simulink model "Copy_of_ModeStatAndRsp"  (R2018b)
settings: Solver=FixedStepDiscrete  StartTime=0.0  StopTime=10.0  FixedStep=0.01  RelTol=1e-3
undefined symbols (not defined in the file): c_RecvL, c_RecvLR, c_RecvR, IfVeSMSeStNumConfig, KeSMSbMdChime2Enable_Val, KeSMSbSRSPosNumConfig_Val, KeSMSuChmReqDurnTm_Val, KeSMSuChmReqIntlTm_Val, KeSMSuRspStatHldTm_Val, MdRspLocal1, MdTp1, ModeNum, PowerMode1, SrcReqTp1, srsconvert
libraries: RspLib x47, simulink x1
(part 6 of 8)

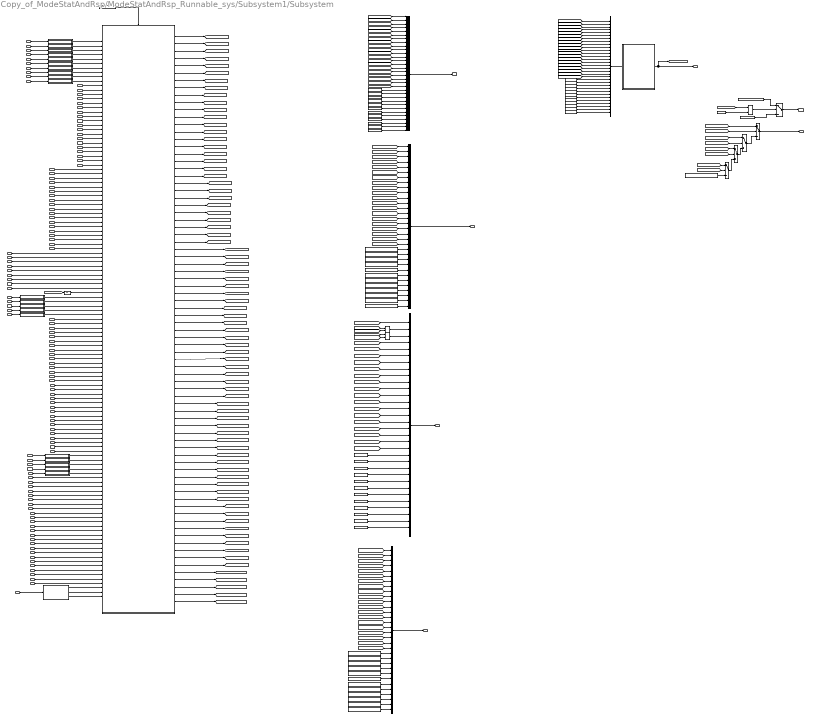
== system Copy_of_ModeStatAndRsp/ModeStatAndRsp_Runnable_sys/Subsystem1/Subsystem ==
  note: **信号已使用不被使用，暂时保留
  acsExtMdReq : Inport
  acsEntyMdReq : Inport  Port=2
  LtVipMdReq : Inport  Port=3
  RtVipMdReq : Inport  Port=4
  AllVipMdReq : Inport  Port=5
  LtLugMdReq : Inport  Port=6
  RtLugMdReq : Inport  Port=7
  AllLugMdReq : Inport  Port=8
  LtRcvyMdReq : Inport  Port=9
  RtRcvyMdReq : Inport  Port=10
  CommCond : Inport  Port=11
  CommExitCond : Inport  Port=12
  CommExitCondwithSpeed : Inport  Port=13
  isAcsMdEntryDoneOK : Inport  Port=14
  isAcsMdExtDoneOK : Inport  Port=15
  isLfLugDoneOK : Inport  Port=16
  isLfRecoveryDoneOK : Inport  Port=17
  isLfVipDoneOK : Inport  Port=18
  isRtLugDoneOK : Inport  Port=19
  isRtRecoveryDoneOK : Inport  Port=20
  isRtVipDoneOK : Inport  Port=21
  isAcsMdEntryDoneFailed : Inport  Port=22
  isAcsMdExtDoneFailed : Inport  Port=23
  isLfLugDoneFailed : Inport  Port=24
  isLfRecoveryDoneFailed : Inport  Port=25
  isLfVipDoneFailed : Inport  Port=26
  isRtLugDoneFailed : Inport  Port=27
  isRtRecoveryDoneFailed : Inport  Port=28
  isRtVipDoneFailed : Inport  Port=29
  SwIntAcsEnty : Inport  Port=30
  SwIntAcsExt : Inport  Port=31
  SwIntLfVip : Inport  Port=32
  SwIntRtVip : Inport  Port=33
  SwIntLfLug : Inport  Port=34
  SwIntRtLug : Inport  Port=35
  SwIntLfRcvy : Inport  Port=36
  SwIntRtRcvy : Inport  Port=37
  SwIntAllLug : Inport  Port=38
  SoftIntAcsExt : Inport  Port=39
  SoftIntAcsEnty : Inport  Port=40
  SoftIntLfVip : Inport  Port=41
  SoftIntRtVip : Inport  Port=42
  SoftIntLfLug : Inport  Port=43
  SoftIntRtLug : Inport  Port=44
  SoftIntLfRcvy : Inport  Port=45
  SoftIntRtRcvy : Inport  Port=46
  SoftIntAllVip : Inport  Port=47
  SoftIntAllLug : Inport  Port=48
  acsExtMdSrcTp : Inport  Port=49
  acsEntyMdSrcTp : Inport  Port=50
  LtVipSrcReqTp : Inport  Port=51
  RtVipSrcReqTp : Inport  Port=52
  LtLugSrcReqTp : Inport  Port=53
  RtLugSrcReqTp : Inport  Port=54
  LtRcvySrcReqTp : Inport  Port=55
  RtRcvySrcReqTp : Inport  Port=56
  AllLugSrcReqTp_Val : Inport  Port=57
  StNumConfig : Inport  Port=58
  INTMMdReq : Inport  Port=59
  LfFamlyReq : Inport  Port=60
  LfLyMdReq : Inport  Port=61
  RtFamlyMdReq : Inport  Port=62
  RtLyMdReq : Inport  Port=63
  INTMSrcReqTp : Inport  Port=64
  LfFamlySrcReqTp : Inport  Port=65
  LfLySrcReqTp : Inport  Port=66
  RtFamlySrcReqTp : Inport  Port=67
  RtLySrcReqTp : Inport  Port=68
  SoftIntINTM : Inport  Port=69
  SoftIntLfFamly : Inport  Port=70
  SoftIntLfLy : Inport  Port=71
  SoftIntRtFamly : Inport  Port=72
  SoftIntRtLy : Inport  Port=73
  SwIntINTM : Inport  Port=74
  SwIntLfFamly : Inport  Port=75
  SwIntLfLy : Inport  Port=76
  SwIntRtFamly : Inport  Port=77
  SwIntRtLy : Inport  Port=78
  isINTMDoneOK : Inport  Port=79
  isFamlyLDoneOK : Inport  Port=80
  isFamlyRDoneOK : Inport  Port=81
  isLfLyDoneOK : Inport  Port=82
  isRtLyDoneOK : Inport  Port=83
  isINTMDoneFailed : Inport  Port=84
  isFamlyLDoneFailed : Inport  Port=85
  isFamlyRDoneFailed : Inport  Port=86
  isLfLyDoneFailed : Inport  Port=87
  isRtLyDoneFailed : Inport  Port=88
  AllVipSrcReqTp : Inport  Port=89
  LugMdLtAvl_Val_read : Inport  Port=90
  LugMdRtAvl_Val_read : Inport  Port=91
  VipMdLtAvl_Val_read : Inport  Port=92
  VipMdRtAvl_Val_read : Inport  Port=93
  SwIntAllVip : Inport  Port=94
  IntimacyRtMdReq_Val_read : Inport  Port=95
  IntimacyRtMdSrcTp_Val_read : Inport  Port=96
  isINTMRDoneFailed_Val_read : Inport  Port=97
  isINTMRDoneOK_Val_read : Inport  Port=98
  isLgrstCloseLDoneFailed_Val_read : Inport  Port=99
  isLgrstCloseLDoneOK_Val_read : Inport  Port=100
  isLgrstCloseRDoneFailed_Val_read : Inport  Port=101
  isLgrstCloseRDoneOK_Val_read : Inport  Port=102
  isLgrstOpenLDoneFailed_Val_read : Inport  Port=103
  isLgrstOpenLDoneOK_Val_read : Inport  Port=104
  isLgrstOpenRDoneFailed_Val_read : Inport  Port=105
  isLgrstOpenRDoneOK_Val_read : Inport  Port=106
  LgrstCloseLtMdReq_Val_read : Inport  Port=107
  LgrstCloseLtSrcReqTp_Val_read : Inport  Port=108
  LgrstCloseRtMdReq_Val_read : Inport  Port=109
  LgrstCloseRtSrcReqTp_Val_read : Inport  Port=110
  LgrstOpenLtMdReq_Val_read : Inport  Port=111
  LgrstOpenLtSrcReqTp_Val_read : Inport  Port=112
  LgrstOpenRtMdReq_Val_read : Inport  Port=113
  LgrstOpenRtSrcReqTp_Val_read : Inport  Port=114
  SoftIntIntimacyRt_Val_read : Inport  Port=115
  SoftIntLgrstCloseLt_Val_read : Inport  Port=116
  SoftIntLgrstCloseRt_Val_read : Inport  Port=117
  SoftIntLgrstOpenLt_Val_read : Inport  Port=118
  SoftIntLgrstOpenRt_Val_read : Inport  Port=119
  SwIntIntimacyRt_Val_read : Inport  Port=120
  SwIntLgrstCloseLt_Val_read : Inport  Port=121
  SwIntLgrstCloseRt_Val_read : Inport  Port=122
  SwIntLgrstOpenLt_Val_read : Inport  Port=123
  SwIntLgrstOpenRt_Val_read : Inport  Port=124
  Bus Creator{,1,3..4} (4 alike) : BusCreator  Inputs=32
  Chart : Stateflow chart  TreatAsAtomicUnit=on
  Chart2 : Stateflow chart  TreatAsAtomicUnit=on
  Constant{7,9..18,36..37} (13 alike) : Constant  Value=SrcReqTp1.SrcReqTp_None  OutDataTypeStr=Enum:SrcReqTp1
  Constant{19..30} (12 alike) : Constant  Description=_SGMK226P2.FCMD.000_369_  Value=0  OutDataTypeStr=boolean
  Constant3 : Constant  Value=MdTp1.MdTp_EzeEntry  OutDataTypeStr=Enum:MdTp1
  Constant{38..49} (12 alike) : Constant  Value=MdRspLocal1.MdRsp_None  OutDataTypeStr=Enum: MdRspLocal1
  Constant5 : Constant  Value=0  OutDataTypeStr=uint32
  Constant{56..67,73..84} (24 alike) : Constant  Value=0  OutDataTypeStr=boolean
  Constant6 : Constant  Value=MdTp1.MdTp_None  OutDataTypeStr=Enum:MdTp1
  Function-Call Generator : simulink/Ports & Subsystems/Function-Call Generator  sample_time=-1  numberOfIterations=2
  HasChangeToTrue : Subsystem
  HasChangeToTrue1 : Subsystem
  HasChangeToTrue10 : Subsystem
  HasChangeToTrue11 : Subsystem
  HasChangeToTrue12 : Subsystem
  HasChangeToTrue13 : Subsystem
  HasChangeToTrue14 : Subsystem
  HasChangeToTrue15 : Subsystem
  HasChangeToTrue16 : Subsystem
  HasChangeToTrue17 : Subsystem
  HasChangeToTrue18 : Subsystem
  HasChangeToTrue19 : Subsystem
  HasChangeToTrue2 : Subsystem
  HasChangeToTrue3 : Subsystem
  HasChangeToTrue4 : Subsystem
  HasChangeToTrue5 : Subsystem
  HasChangeToTrue6 : Subsystem
  HasChangeToTrue7 : Subsystem
  HasChangeToTrue8 : Subsystem
  HasChangeToTrue9 : Subsystem
  Mux11 : Mux  Inputs=32
  OR : Logic  Operator=OR  AllPortsSameDT=off  OutDataTypeStr=boolean
  OR1 : Logic  Operator=OR  AllPortsSameDT=off  OutDataTypeStr=boolean
  Relational Operator : RelationalOperator  Operator=>  OutDataTypeStr=boolean  RndMeth=Simplest
  StNumChk : Subsystem
  Switch{,1..4} (5 alike) : Switch  Criteria=u2 > Threshold
  Unit Delay9 : UnitDelay  SampleTime=-1
  oModeState : Outport
  ModeSrcTpLt : Outport  Port=2  VectorParamsAs1DForOutWhenUnconnected=on
  ModeState32 : Outport  Port=3
  MdStateBus : Outport  Port=4
  MdBsy : Outport  Port=5
  MdSrcTp : Outport  Port=6
  MdRsp : Outport  Port=7
  wires:
  SwIntRtVip/1 -> Chart/33(SwIntRtVip)
  isRtLugDoneOK/1 -> Chart/19(iIsRtLugDoneOK)
  SoftIntAcsEnty/1 -> Chart/40(SoftIntAcsEnty)
  SoftIntLfRcvy/1 -> Chart/45(SoftIntLfRcvy)
  SoftIntRtRcvy/1 -> Chart/46(SoftIntRtRcvy)
  isRtRecoveryDoneFailed/1 -> Chart/28(iIsRtRecoveryDoneFailed)
  isAcsMdExtDoneFailed/1 -> Chart/23(iIsAcsMdExtDoneFailed)
  isAcsMdEntryDoneOK/1 -> Chart/14(iIsAcsMdEntryDoneOK)
  SwIntAcsExt/1 -> Chart/31(SwIntAcsExt)
  SoftIntRtLug/1 -> Chart/44(SoftIntRtLug)
  SoftIntRtVip/1 -> Chart/42(SoftIntRtVip)
  isRtRecoveryDoneOK/1 -> Chart/20(iIsRtRecoveryDoneOK)
  SoftIntAllLug/1 -> Chart/48(SoftIntAllLug)
  isAcsMdEntryDoneFailed/1 -> Chart/22(iIsAcsMdEntryDoneFailed)
  SwIntRtRcvy/1 -> Chart/37(SwIntRtRcvy)
  isLfLugDoneFailed/1 -> Chart/24(iIsLtLugDoneFailed)
  CommExitCond/1 -> Chart/12(CommExitCond)
  isLfVipDoneOK/1 -> Chart/18(iIsLtVipDoneOK)
  CommCond/1 -> Chart/11(CommCond)
  SwIntRtLug/1 -> Chart/35(SwIntRtLug)
  SoftIntAllVip/1 -> Chart/47(SoftIntAllVip)
  isAcsMdExtDoneOK/1 -> Chart/15(iIsAcsMdExtDoneOK)
  isLfLugDoneOK/1 -> Chart/16(iIsLtLugDoneOK)
  SoftIntAcsExt/1 -> Chart/39(SoftIntAcsExt)
  SwIntAllLug/1 -> Chart/38(SwIntAllLug)
  isLfRecoveryDoneOK/1 -> Chart/17(iIsLtRecoveryDoneOK)
  isRtVipDoneOK/1 -> Chart/21(iIsRtVipDoneOK)
  isRtLugDoneFailed/1 -> Chart/27(iIsRtLugDoneFailed)
  SoftIntLfVip/1 -> Chart/41(SoftIntLfVip)
  isLfRecoveryDoneFailed/1 -> Chart/25(iIsLtRecoveryDoneFailed)
  SwIntLfRcvy/1 -> Chart/36(SwIntLfRcvy)
  isLfVipDoneFailed/1 -> Chart/26(iIsLtVipDoneFailed)
  isRtVipDoneFailed/1 -> Chart/29(iIsRtVipDoneFailed)
  SwIntLfLug/1 -> Chart/34(SwIntLfLug)
  SoftIntLfLug/1 -> Chart/43(SoftIntLfLug)
  SwIntAcsEnty/1 -> Chart/30(SwIntAcsEnty)
  SwIntLfVip/1 -> Chart/32(SwIntLfVip)
  CommExitCondwithSpeed/1 -> Chart/13(CommExitCondwithSpeed)
  [LgrstOpenR_En] -> Mux11/18
  Mux11/1 -> Chart2/1(ModeArray)
  Constant20/1 -> Mux11/22
  Constant26/1 -> Mux11/28
  [LgrstCloseL_En] -> Mux11/17
  [RecoveryR_En] -> Mux11/13
  [FAMLY_R_En] -> Mux11/6
  [LgrstCloseR_En] -> Mux11/19
  [INTM_En] -> Mux11/5
  [INTMR_En] -> Mux11/20
  [LgrstOpenL_En] -> Mux11/16
  Constant29/1 -> Mux11/31
  [RecoveryL_En] -> Mux11/11
  Constant28/1 -> Mux11/30
  Constant27/1 -> Mux11/29
  [VIPR_En] -> Mux11/12
  [LugL_En] -> Mux11/8
  [VIPAll_En] -> Mux11/2
  Constant22/1 -> Mux11/24
  Constant24/1 -> Mux11/26
  [LyL_En] -> Mux11/14
  [EZE_En] -> Mux11/1
  [LugAll_En] -> Mux11/3
  [FAMLY_L_En] -> Mux11/7
  [LugR_En] -> Mux11/9
  Constant30/1 -> Mux11/32
  Constant23/1 -> Mux11/25
  Constant19/1 -> Mux11/21
  [EZQ_En] -> Mux11/4
  [VIPL_En] -> Mux11/10
  Constant25/1 -> Mux11/27
  Constant21/1 -> Mux11/23
  [LyR_En] -> Mux11/15
  Chart/11(RecoveryL_En) -> [RecoveryL_En]
  Chart/10(VIPL_En) -> [VIPL_En]
  Chart/12(VIPR_En) -> [VIPR_En]
  Chart/9(LugR_En) -> [LugR_En]
  Chart/13(RecoveryR_En) -> [RecoveryR_En]
  Chart/8(LugL_En) -> [LugL_En]
  Chart/14(LyL_En) -> [LyL_En]
  Chart/7(FAMLY_L_En) -> [FAMLY_L_En]
  Chart/15(LyR_En) -> [LyR_En]
  Chart/6(FAMLY_R_En) -> [FAMLY_R_En]
  Chart/5(INTM_En) -> [INTM_En]
  Chart/4(EZQ_En) -> [EZQ_En]
  Chart/3(LugAll_En) -> [LugAll_En]
  Chart/2(VIPAll_En) -> [VIPAll_En]
  Chart2/1(ModeState32) -> [ModeState32], ModeState32/1
  [ModeState32] -> Relational Operator/1
  Constant5/1 -> Relational Operator/2
  Relational Operator/1 -> Switch/2
  Constant3/1 -> Switch/1
  Switch/1 -> oModeState/1
  Constant6/1 -> Switch/3
  Chart/21(ModeSrcTpAllLug) -> [ModeSrcTpAllLug]
  Chart/22(ModeSrcTpEZE) -> [ModeSrcTpEZE]
  Chart/23(ModeSrcTpEZQ) -> [ModeSrcTpEZQ]
  Chart/24(ModeSrcTpLtLug) -> [ModeSrcTpLtLug]
  Chart/25(ModeSrcTpLtRecovery) -> [ModeSrcTpLtRecovery]
  Chart/26(ModeSrcTpLtVIP) -> [ModeSrcTpLtVIP]
  Chart/27(ModeSrcTpRtLug) -> [ModeSrcTpRtLug]
  Chart/28(ModeSrcTpRtRecovery) -> [ModeSrcTpRtRecovery]
  Chart/29(ModeSrcTpRtVIP) -> [ModeSrcTpRtVIP]
  Chart/1(EZE_En) -> [EZE_En]
  [ModeState32] -> Unit Delay9/1
  Unit Delay9/1 -> Chart/58(modestate32)
  Switch1/1 -> ModeSrcTpLt/1
  [EZE_En] -> Switch1/2
  [ModeSrcTpEZE] -> Switch1/1
  Switch2/1 -> Switch1/3
  [EZQ_En] -> Switch2/2
  [ModeSrcTpEZQ] -> Switch2/1
  Switch3/1 -> Switch2/3
  [VIPAll_En] -> Switch3/2
  [ModeSrcTpALLVIP] -> Switch3/1
  Switch4/1 -> Switch3/3
  [LugAll_En] -> Switch4/2
  [ModeSrcTpAllLug] -> Switch4/1
  Constant7/1 -> Switch4/3
  SoftIntINTM/1 -> Chart/64(SoftIntINTM)
  SoftIntLfFamly/1 -> Chart/65(SoftIntLfFamly)
  SoftIntLfLy/1 -> Chart/66(SoftIntLfLy)
  SoftIntRtFamly/1 -> Chart/67(SoftIntRtFamly)
  SoftIntRtLy/1 -> Chart/68(SoftIntRtLy)
  SwIntINTM/1 -> Chart/69(SwIntINTM)
  SwIntLfFamly/1 -> Chart/70(SwIntLfFamly)
  SwIntLfLy/1 -> Chart/71(SwIntLfLy)
  SwIntRtFamly/1 -> Chart/72(SwIntRtFamly)
  SwIntRtLy/1 -> Chart/73(SwIntRtLy)
  isINTMDoneOK/1 -> Chart/74(isINTMDoneOK)
  isFamlyLDoneOK/1 -> Chart/75(isFamlyLDoneOK)
  isFamlyRDoneOK/1 -> Chart/76(isFamlyRDoneOK)
  isLfLyDoneOK/1 -> Chart/77(isLfLyDoneOK)
  isRtLyDoneOK/1 -> Chart/78(isRtLyDoneOK)
  isINTMDoneFailed/1 -> Chart/79(isINTMDoneFailed)
  isFamlyLDoneFailed/1 -> Chart/80(isFamlyLDoneFailed)
  isFamlyRDoneFailed/1 -> Chart/81(isFamlyRDoneFailed)
  isLfLyDoneFailed/1 -> Chart/82(isLfLyDoneFailed)
  isRtLyDoneFailed/1 -> Chart/83(isRtLyDoneFailed)
  Chart/50(ModeSrcTpALLVIP) -> [ModeSrcTpALLVIP]
  Chart/52(EZQStBsy) -> [EZQStBsy]
  Chart/51(EZEStBsy) -> [EZEStBsy]
  Chart/53(VIPLStBsy) -> [VIPLStBsy]
  Chart/54(VIPRStBsy) -> [VIPRStBsy]
  Chart/55(RecoveryLStBsy) -> [RecoveryLStBsy]
  Chart/56(RecoveryRStBsy) -> [RecoveryRStBsy]
  Chart/57(LugLStBsy) -> [LugLStBsy]
  Chart/58(LugRStBsy) -> [LugRStBsy]
  Chart/59(FamlyLBsy) -> [FamilyLStBsy]
  Chart/60(FamlyRBsy) -> [FamilyRStBsy]
  Chart/61(INTMBsy) -> [INTMBsy]
  Chart/62(LyLBsy) -> [LyLBsy]
  Chart/63(LyRBsy) -> [LyRBsy]
  LugMdLtAvl_Val_read/1 -> Chart/90(LugMdLtAvl)
  LugMdRtAvl_Val_read/1 -> Chart/91(LugMdRtAvl)
  VipMdLtAvl_Val_read/1 -> Chart/92(VipMdLtAvl)
  VipMdRtAvl_Val_read/1 -> Chart/93(VipMdRtAvl)
  SwIntAllVip/1 -> Chart/94(SwIntAllVip)
  Function-Call Generator/1 -> Chart/Trigger
  acsExtMdReq/1 -> HasChangeToTrue/1(In1)
  acsEntyMdReq/1 -> HasChangeToTrue1/1(In1)
  LtVipMdReq/1 -> HasChangeToTrue2/1(In1)
  RtVipMdReq/1 -> HasChangeToTrue3/1(In1)
  AllVipMdReq/1 -> HasChangeToTrue4/1(In1)
  LtLugMdReq/1 -> HasChangeToTrue5/1(In1)
  RtLugMdReq/1 -> HasChangeToTrue6/1(In1)
  AllLugMdReq/1 -> HasChangeToTrue7/1(In1)
  LtRcvyMdReq/1 -> HasChangeToTrue8/1(In1)
  RtRcvyMdReq/1 -> HasChangeToTrue9/1(In1)
  acsExtMdSrcTp/1 -> Chart/49(acsExtMdSrcTp)
  acsEntyMdSrcTp/1 -> Chart/50(acsEntyMdSrcTp)
  LtVipSrcReqTp/1 -> Chart/51(LtVipSrcReqTp)
  RtVipSrcReqTp/1 -> Chart/52(RtVipSrcReqTp)
  LtLugSrcReqTp/1 -> Chart/53(LtLugSrcReqTp)
  RtLugSrcReqTp/1 -> Chart/54(RtLugSrcReqTp)
  LtRcvySrcReqTp/1 -> Chart/55(LtRcvySrcReqTp)
  RtRcvySrcReqTp/1 -> Chart/56(RtRcvySrcReqTp)
  AllLugSrcReqTp_Val/1 -> Chart/57(AllLugSrcReqTp)
  INTMMdReq/1 -> HasChangeToTrue10/1(In1)
  LfFamlyReq/1 -> HasChangeToTrue11/1(In1)
  LfLyMdReq/1 -> HasChangeToTrue12/1(In1)
  RtFamlyMdReq/1 -> HasChangeToTrue13/1(In1)
  RtLyMdReq/1 -> HasChangeToTrue14/1(In1)
  INTMSrcReqTp/1 -> Chart/84(INTMSrcReqTp)
  LfFamlySrcReqTp/1 -> Chart/85(LfFamlySrcReqTp)
  LfLySrcReqTp/1 -> Chart/86(LfLySrcReqTp)
  RtFamlySrcReqTp/1 -> Chart/87(RtFamlySrcReqTp)
  RtLySrcReqTp/1 -> Chart/88(RtLySrcReqTp)
  AllVipSrcReqTp/1 -> Chart/89(AllVipSrcReqTp)
  HasChangeToTrue/1(Out1) -> Chart/1(acsExtMdReq)
  HasChangeToTrue1/1(Out1) -> Chart/2(acsEntyMdReq)
  HasChangeToTrue2/1(Out1) -> Chart/3(LtVipMdReq)
  HasChangeToTrue3/1(Out1) -> Chart/4(RtVipMdReq)
  HasChangeToTrue4/1(Out1) -> Chart/5(AllVipMdReq)
  HasChangeToTrue5/1(Out1) -> Chart/6(LtLugMdReq)
  HasChangeToTrue6/1(Out1) -> Chart/7(RtLugMdReq)
  HasChangeToTrue7/1(Out1) -> Chart/8(AllLugMdReq)
  HasChangeToTrue8/1(Out1) -> Chart/9(LtRcvyMdReq)
  HasChangeToTrue9/1(Out1) -> Chart/10(RtRcvyMdReq)
  HasChangeToTrue10/1(Out1) -> Chart/59(INTMMdReq)
  HasChangeToTrue11/1(Out1) -> Chart/60(LfFamlyMdReq)
  HasChangeToTrue12/1(Out1) -> Chart/61(LfLyMdReq)
  HasChangeToTrue13/1(Out1) -> Chart/62(RtFamlyMdReq)
  HasChangeToTrue14/1(Out1) -> Chart/63(RtLyMdReq)
  Chart/16(LgrstOpenL_En) -> [LgrstOpenL_En]
  Chart/17(LgrstCloseL_En) -> [LgrstCloseL_En]
  Chart/18(LgrstOpenR_En) -> [LgrstOpenR_En]
  Chart/19(LgrstCloseR_En) -> [LgrstCloseR_En]
  Chart/20(INTMR_En) -> [INTMR_En]
  IntimacyRtMdReq_Val_read/1 -> HasChangeToTrue15/1(In1)
  LgrstCloseLtMdReq_Val_read/1 -> HasChangeToTrue16/1(In1)
  LgrstCloseRtMdReq_Val_read/1 -> HasChangeToTrue17/1(In1)
  LgrstOpenLtMdReq_Val_read/1 -> HasChangeToTrue18/1(In1)
  LgrstOpenRtMdReq_Val_read/1 -> HasChangeToTrue19/1(In1)
  IntimacyRtMdSrcTp_Val_read/1 -> Chart/100(INTMRSrcReqTp)
  LgrstCloseLtSrcReqTp_Val_read/1 -> Chart/101(LgrstCloseLtSrcReqTp)
  LgrstCloseRtSrcReqTp_Val_read/1 -> Chart/102(LgrstCloseRtSrcReqTp)
  LgrstOpenLtSrcReqTp_Val_read/1 -> Chart/103(LgrstOpenLtSrcReqTp)
  LgrstOpenRtSrcReqTp_Val_read/1 -> Chart/104(LgrstOpenRtSrcReqTp)
  isINTMRDoneFailed_Val_read/1 -> Chart/105(isINTMRDoneFailed)
  isLgrstCloseLDoneFailed_Val_read/1 -> Chart/106(isLgrstCloseLDoneFailed)
  isLgrstCloseRDoneFailed_Val_read/1 -> Chart/107(isLgrstCloseRDoneFailed)
  isLgrstOpenLDoneFailed_Val_read/1 -> Chart/108(isLgrstOpenLDoneFailed)
  isLgrstOpenRDoneFailed_Val_read/1 -> Chart/109(isLgrstOpenRDoneFailed)
  isINTMRDoneOK_Val_read/1 -> Chart/110(isINTMRDoneOK)
  isLgrstCloseLDoneOK_Val_read/1 -> Chart/111(isLgrstCloseLDoneOK)
  isLgrstCloseRDoneOK_Val_read/1 -> Chart/112(isLgrstCloseRDoneOK)
  isLgrstOpenLDoneOK_Val_read/1 -> Chart/113(isLgrstOpenLDoneOK)
  isLgrstOpenRDoneOK_Val_read/1 -> Chart/114(isLgrstOpenRDoneOK)
  SoftIntIntimacyRt_Val_read/1 -> Chart/115(SoftIntINTMR)
  SoftIntLgrstCloseLt_Val_read/1 -> Chart/116(SoftIntLgrstCloseLt)
  SoftIntLgrstCloseRt_Val_read/1 -> Chart/117(SoftIntLgrstCloseRt)
  SoftIntLgrstOpenLt_Val_read/1 -> Chart/118(SoftIntLgrstOpenLt)
  SoftIntLgrstOpenRt_Val_read/1 -> Chart/119(SoftIntLgrstOpenRt)
  SwIntIntimacyRt_Val_read/1 -> Chart/120(SwIntINTMR)
  SwIntLgrstCloseLt_Val_read/1 -> Chart/121(SwIntLgrstCloseLt)
  SwIntLgrstCloseRt_Val_read/1 -> Chart/122(SwIntLgrstCloseRt)
  SwIntLgrstOpenLt_Val_read/1 -> Chart/123(SwIntLgrstOpenLt)
  SwIntLgrstOpenRt_Val_read/1 -> Chart/124(SwIntLgrstOpenRt)
  HasChangeToTrue15/1(Out1) -> Chart/95(INTMRMdReq)
  HasChangeToTrue16/1(Out1) -> Chart/96(LgrstCloseLtMdReq)
  HasChangeToTrue17/1(Out1) -> Chart/97(LgrstCloseRtMdReq)
  HasChangeToTrue18/1(Out1) -> Chart/98(LgrstOpenLtMdReq)
  HasChangeToTrue19/1(Out1) -> Chart/99(LgrstOpenRtMdReq)
  Chart/78(INTMRBsy) -> [INTMRBsy]
  Chart/77(LgrstCloseRBsy) -> [LgrstCloseRBsy]
  Chart/75(LgrstCloseLBsy) -> [LgrstCloseLBsy]
  Chart/76(LgrstOpenRBsy) -> [LgrstOpenRBsy]
  Chart/74(LgrstOpenLBsy) -> [LgrstOpenLBsy]
  [LgrstCloseR_En] -> Bus Creator3/19  "Md19_En"
  [LgrstOpenL_En] -> Bus Creator3/16  "Md16_En"
  [EZE_En] -> Bus Creator3/1  "Md1_En"
  [LugL_En] -> Bus Creator3/8  "Md8_En"
  Constant67/1 -> Bus Creator3/32  "Md32_En"
  [FAMLY_L_En] -> Bus Creator3/7  "Md7_En"
  [RecoveryR_En] -> Bus Creator3/13  "Md13_En"
  Constant61/1 -> Bus Creator3/26  "Md26_En"
  [FAMLY_R_En] -> Bus Creator3/6  "Md6_En"
  [LgrstOpenR_En] -> Bus Creator3/18  "Md18_En"
  Constant57/1 -> Bus Creator3/22  "Md22_En"
  Constant59/1 -> Bus Creator3/24  "Md24_En"
  Constant56/1 -> Bus Creator3/21  "Md21_En"
  [LyR_En] -> Bus Creator3/15  "Md15_En"
  Constant65/1 -> Bus Creator3/30  "Md30_En"
  Constant64/1 -> Bus Creator3/29  "Md29_En"
  Constant66/1 -> Bus Creator3/31  "Md31_En"
  Constant62/1 -> Bus Creator3/27  "Md27_En"
  Constant58/1 -> Bus Creator3/23  "Md23_En"
  [VIPAll_En] -> Bus Creator3/2  "Md2_En"
  [INTMR_En] -> Bus Creator3/20  "Md20_En"
  [VIPL_En] -> Bus Creator3/10  "Md10_En"
  [LgrstCloseL_En] -> Bus Creator3/17  "Md17_En"
  [LyL_En] -> Bus Creator3/14  "Md14_En"
  [RecoveryL_En] -> Bus Creator3/11  "Md11_En"
  [LugR_En] -> Bus Creator3/9  "Md9_En"
  Constant60/1 -> Bus Creator3/25  "Md25_En"
  [LugAll_En] -> Bus Creator3/3  "Md3_En"
  [INTM_En] -> Bus Creator3/5  "Md5_En"
  [EZQ_En] -> Bus Creator3/4  "Md4_En"
  Constant63/1 -> Bus Creator3/28  "Md28_En"
  [VIPR_En] -> Bus Creator3/12  "Md12_En"
  Bus Creator3/1 -> MdStateBus/1
  Constant76/1 -> Bus Creator4/24  "Md24Exit"
  [LyRBsy] -> Bus Creator4/15  "Md15Exit"
  Constant82/1 -> Bus Creator4/30  "Md30Exit"
  Constant78/1 -> Bus Creator4/26  "Md26Exit"
  Constant80/1 -> Bus Creator4/28  "Md28Exit"
  [EZEStBsy] -> Bus Creator4/1  "Md1Exit"
  Constant79/1 -> Bus Creator4/27  "Md27Exit"
  [LugLStBsy] -> Bus Creator4/8  "Md8Exit"
  Constant81/1 -> Bus Creator4/29  "Md29Exit"
  Constant77/1 -> Bus Creator4/25  "Md25Exit"
  Constant75/1 -> Bus Creator4/23  "Md23Exit"
  [INTMRBsy] -> Bus Creator4/20  "Md20Exit"
  Constant73/1 -> Bus Creator4/21  "Md21Exit"
  [LgrstCloseRBsy] -> Bus Creator4/19  "Md19Exit"
  [FamilyRStBsy] -> Bus Creator4/6  "Md6Exit"
  [LyLBsy] -> Bus Creator4/14  "Md14Exit"
  Constant83/1 -> Bus Creator4/31  "Md31Exit"
  [FamilyLStBsy] -> Bus Creator4/7  "Md7Exit"
  [LugLStBsy] -> OR1/1
  [RecoveryRStBsy] -> Bus Creator4/13  "Md13Exit"
  [EZQStBsy] -> Bus Creator4/4  "Md4Exit"
  [LugRStBsy] -> Bus Creator4/9  "Md9Exit"
  [LgrstCloseLBsy] -> Bus Creator4/17  "Md17Exit"
  OR1/1 -> Bus Creator4/3  "Md3Exit"
  Bus Creator4/1 -> MdBsy/1  "MdBsy"
  [LgrstOpenRBsy] -> Bus Creator4/18  "Md18Exit"
  [RecoveryLStBsy] -> Bus Creator4/11  "Md11Exit"
  [INTMBsy] -> Bus Creator4/5  "Md5Exit"
  [LugRStBsy] -> OR1/2
  Constant84/1 -> Bus Creator4/32  "Md32Exit"
  OR/1 -> Bus Creator4/2  "Md2Exit"
  [VIPRStBsy] -> Bus Creator4/12  "Md12Exit"
  [VIPLStBsy] -> OR/1
  [VIPRStBsy] -> OR/2
  [LgrstOpenLBsy] -> Bus Creator4/16  "Md16Exit"
  [VIPLStBsy] -> Bus Creator4/10  "Md10Exit"
  Constant74/1 -> Bus Creator4/22  "Md22Exit"
  Chart/64(ModeSrcTpLgrstOpenL) -> [ModeSrcTpLgrstOpenL]
  Chart/65(ModeSrcTpLgrstCloseL) -> [ModeSrcTpLgrstCloseL]
  Chart/66(ModeSrcTpLgrstOpenR) -> [ModeSrcTpLgrstOpenR]
  Chart/67(ModeSrcTpLgrstCloseR) -> [ModeSrcTpLgrstCloseR]
  Chart/68(ModeSrcTpINTMR) -> [ModeSrcTpINTMR]
  Chart/69(oModeRspLgrstOpenL) -> [ModeRspLgrstOpenL]
  Chart/70(oModeRspLgrstCloseL) -> [ModeRspLgrstCloseL]
  Chart/71(oModeRspLgrstOpenR) -> [ModeRspLgrstOpenR]
  Chart/72(oModeRspLgrstCloseR) -> [ModeRspLgrstCloseR]
  Chart/73(oModeRspINTMR) -> [ModeRspINTMR]
  Chart/30(oModeRspEZE) -> [ModeRspEZE]
  Chart/31(oModeRspEZQ) -> [ModeRspEZQ]
  Chart/32(oModeRspLtLug) -> [ModeRspLtLug]
  Chart/38(oModeRspVIPALL) -> [ModeRspVIPALL]
  Chart/33(oModeRspLtRecovery) -> [ModeRspLtRecovery]
  Chart/34(oModeRspLtVIP) -> [ModeRspLtVIP]
  Chart/35(oModeRspRtLug) -> [ModeRspRtLug]
  Chart/36(oModeRspRtRecovery) -> [ModeRspRtRecovery]
  Chart/37(oModeRspRtVIP) -> [ModeRspRtVIP]
  Chart/39(oModeRspLugALL) -> [ModeRspLugALL]
  Chart/40(ModeSrcTpINTM) -> [ModeSrcTpINTM]
  Chart/41(ModeSrcTpLfFamly) -> [ModeSrcTpLfFamly]
  Chart/42(ModeSrcTpLfLy) -> [ModeSrcTpLfLy]
  Chart/43(ModeSrcTpRtFamly) -> [ModeSrcTpRtFamly]
  Chart/44(ModeSrcTpRtLy) -> [ModeSrcTpRtLy]
  Chart/46(oModeRspLfFamly) -> [ModeRspLfFamly]
  Chart/47(oModeRspLfLy) -> [ModeRspLfLy]
  Chart/48(oModeRspRtFamly) -> [ModeRspRtFamly]
  Chart/49(oModeRspRtLy) -> [ModeRspRtLy]
  Chart/45(oModeRspINTM) -> [ModeRspINTM]
  [ModeSrcTpLtLug] -> Bus Creator/8  "Md8SrcTp"
  [ModeSrcTpLgrstCloseL] -> Bus Creator/17  "Md17SrcTp"
  Constant14/1 -> Bus Creator/29  "Md29SrcTp"
  Constant12/1 -> Bus Creator/25  "Md25SrcTp"
  [ModeSrcTpRtLug] -> Bus Creator/9  "Md9SrcTp"
  [ModeSrcTpLgrstOpenR] -> Bus Creator/18  "Md18SrcTp"
  [ModeSrcTpRtFamly] -> Bus Creator/6  "Md6SrcTp"
  [ModeSrcTpLfLy] -> Bus Creator/14  "Md14SrcTp"
  [ModeSrcTpLgrstOpenL] -> Bus Creator/16  "Md16SrcTp"
  [ModeSrcTpINTM] -> Bus Creator/5  "Md5SrcTp"
  [ModeSrcTpEZQ] -> Bus Creator/4  "Md4SrcTp"
  [ModeSrcTpRtLy] -> Bus Creator/15  "Md15SrcTp"
  Constant18/1 -> Bus Creator/31  "Md31SrcTp"
  Constant11/1 -> Bus Creator/24  "Md24SrcTp"
  Constant17/1 -> Bus Creator/26  "Md26SrcTp"
  Constant10/1 -> Bus Creator/23  "Md23SrcTp"
  Constant15/1 -> Bus Creator/30  "Md30SrcTp"
  Constant13/1 -> Bus Creator/28  "Md28SrcTp"
  [ModeSrcTpLtVIP] -> Bus Creator/10  "Md10SrcTp"
  Constant9/1 -> Bus Creator/32  "Md32SrcTp"
  [ModeSrcTpINTMR] -> Bus Creator/20  "Md20SrcTp"
  Constant37/1 -> Bus Creator/21  "Md21SrcTp"
  [ModeSrcTpALLVIP] -> Bus Creator/2  "Md2SrcTp"
  [ModeSrcTpLgrstCloseR] -> Bus Creator/19  "Md19SrcTp"
  Constant16/1 -> Bus Creator/27  "Md27SrcTp"
  [ModeSrcTpLtRecovery] -> Bus Creator/11  "Md11SrcTp"
  [ModeSrcTpEZE] -> Bus Creator/1  "Md1SrcTp"
  Bus Creator/1 -> MdSrcTp/1  "MdSrcTp"
  [ModeSrcTpLfFamly] -> Bus Creator/7  "Md7SrcTp"
  [ModeSrcTpRtRecovery] -> Bus Creator/13  "Md13SrcTp"
  Constant36/1 -> Bus Creator/22  "Md22SrcTp"
  [ModeSrcTpRtVIP] -> Bus Creator/12  "Md12SrcTp"
  [ModeSrcTpAllLug] -> Bus Creator/3  "Md3SrcTp"
  Bus Creator1/1 -> MdRsp/1  "MdRsp"
  [ModeRspRtRecovery] -> Bus Creator1/13  "Md13Rsp"
  [ModeRspRtLy] -> Bus Creator1/15  "Md15Rsp"
  Constant39/1 -> Bus Creator1/22  "Md22Rsp"
  [ModeRspLgrstOpenR] -> Bus Creator1/18  "Md18Rsp"
  Constant47/1 -> Bus Creator1/30  "Md30Rsp"
  [ModeRspEZQ] -> Bus Creator1/4  "Md4Rsp"
  Constant44/1 -> Bus Creator1/27  "Md27Rsp"
  [ModeRspLgrstOpenL] -> Bus Creator1/16  "Md16Rsp"
  [ModeRspLtVIP] -> Bus Creator1/10  "Md10Rsp"
  [ModeRspLtRecovery] -> Bus Creator1/11  "Md11Rsp"
  Constant46/1 -> Bus Creator1/29  "Md29Rsp"
  [ModeRspLugALL] -> Bus Creator1/3  "Md3Rsp"
  [ModeRspLfFamly] -> Bus Creator1/7  "Md7Rsp"
  [ModeRspLtLug] -> Bus Creator1/8  "Md8Rsp"
  Constant49/1 -> Bus Creator1/32  "Md32Rsp"
  [ModeRspINTM] -> Bus Creator1/5  "Md5Rsp"
  Constant42/1 -> Bus Creator1/25  "Md25Rsp"
  Constant43/1 -> Bus Creator1/26  "Md26Rsp"
  Constant45/1 -> Bus Creator1/28  "Md28Rsp"
  [ModeRspINTMR] -> Bus Creator1/20  "Md20Rsp"
  [ModeRspLgrstCloseR] -> Bus Creator1/19  "Md19Rsp"
  Constant41/1 -> Bus Creator1/24  "Md24Rsp"
  Constant40/1 -> Bus Creator1/23  "Md23Rsp"
  [ModeRspRtLug] -> Bus Creator1/9  "Md9Rsp"
  Constant38/1 -> Bus Creator1/21  "Md21Rsp"
  [ModeRspRtFamly] -> Bus Creator1/6  "Md6Rsp"
  [ModeRspRtVIP] -> Bus Creator1/12  "Md12Rsp"
  [ModeRspEZE] -> Bus Creator1/1  "Md1Rsp"
  Constant48/1 -> Bus Creator1/31  "Md31Rsp"
  [ModeRspVIPALL] -> Bus Creator1/2  "Md2Rsp"
  [ModeRspLfLy] -> Bus Creator1/14  "Md14Rsp"
  [ModeRspLgrstCloseL] -> Bus Creator1/17  "Md17Rsp"
  StNumConfig/1 -> StNumChk/1(StNumConfig)
  StNumChk/1(is7s) -> Chart/125(is7s)
  StNumChk/2(is6s) -> Chart/126(is6s)
  StNumChk/3(is4s) -> Chart/127(is4s)

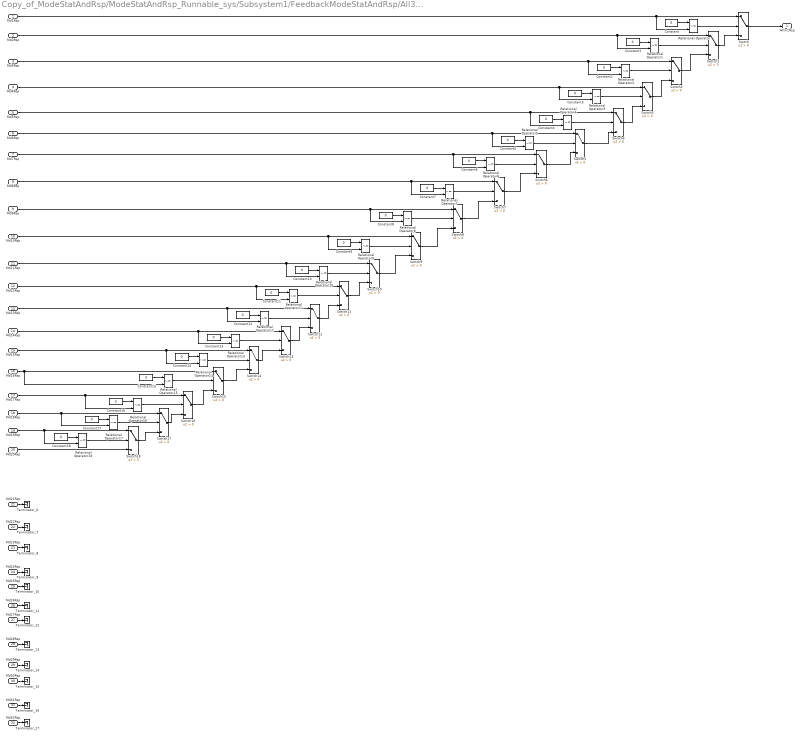
== system Copy_of_ModeStatAndRsp/ModeStatAndRsp_Runnable_sys/Subsystem1/FeedbackModeStatAndRsp/All32in1 ==
  Md1Rsp : Inport
  Md2Rsp : Inport  Port=2
  Md3Rsp : Inport  Port=3
  Md4Rsp : Inport  Port=4
  Md5Rsp : Inport  Port=5
  Md6Rsp : Inport  Port=6
  Md7Rsp : Inport  Port=7
  Md8Rsp : Inport  Port=8
  Md9Rsp : Inport  Port=9
  Md10Rsp : Inport  Port=10
  Md11Rsp : Inport  Port=11
  Md12Rsp : Inport  Port=12
  Md13Rsp : Inport  Port=13
  Md14Rsp : Inport  Port=14
  Md15Rsp : Inport  Port=15
  Md16Rsp : Inport  Port=16
  Md17Rsp : Inport  Port=17
  Md18Rsp : Inport  Port=18
  Md19Rsp : Inport  Port=19
  Md20Rsp : Inport  Port=20
  Md21Rsp : Inport  Port=21
  Md22Rsp : Inport  Port=22
  Md23Rsp : Inport  Port=23
  Md24Rsp : Inport  Port=24
  Md25Rsp : Inport  Port=25
  Md26Rsp : Inport  Port=26
  Md27Rsp : Inport  Port=27
  Md28Rsp : Inport  Port=28
  Md29Rsp : Inport  Port=29
  Md30Rsp : Inport  Port=30
  Md31Rsp : Inport  Port=31
  Md32Rsp : Inport  Port=32
  Constant{,1..18} (19 alike) : Constant  Value=0  OutDataTypeStr=uint8
  Relational Operator{,1..18} (19 alike) : RelationalOperator  Operator=~=  OutDataTypeStr=boolean  RndMeth=Simplest
  Switch{,1..18} (19 alike) : Switch  Criteria=u2 > Threshold
  Terminator_{6..17} (12 alike) : Terminator
  Allin1Rsp : Outport
  wires:
  Md1Rsp/1 -> Relational Operator/2, Switch/1
  Constant/1 -> Relational Operator/1
  Relational Operator/1 -> Switch/2
  Switch/1 -> Allin1Rsp/1
  Switch1/1 -> Switch/3
  Relational Operator1/1 -> Switch1/2
  Constant1/1 -> Relational Operator1/1
  Md2Rsp/1 -> Relational Operator1/2, Switch1/1
  Md3Rsp/1 -> Relational Operator2/2, Switch2/1
  Constant2/1 -> Relational Operator2/1
  Relational Operator2/1 -> Switch2/2
  Switch2/1 -> Switch1/3
  Switch3/1 -> Switch2/3
  Relational Operator3/1 -> Switch3/2
  Constant3/1 -> Relational Operator3/1
  Md4Rsp/1 -> Relational Operator3/2, Switch3/1
  Md5Rsp/1 -> Relational Operator4/2, Switch4/1
  Constant4/1 -> Relational Operator4/1
  Relational Operator4/1 -> Switch4/2
  Switch4/1 -> Switch3/3
  Relational Operator5/1 -> Switch5/2
  Constant5/1 -> Relational Operator5/1
  Md6Rsp/1 -> Relational Operator5/2, Switch5/1
  Switch5/1 -> Switch4/3
  Switch6/1 -> Switch5/3
  Md7Rsp/1 -> Relational Operator6/2, Switch6/1
  Constant6/1 -> Relational Operator6/1
  Relational Operator6/1 -> Switch6/2
  Relational Operator7/1 -> Switch7/2
  Constant7/1 -> Relational Operator7/1
  Md8Rsp/1 -> Relational Operator7/2, Switch7/1
  Switch7/1 -> Switch6/3
  Switch8/1 -> Switch7/3
  Md9Rsp/1 -> Relational Operator8/2, Switch8/1
  Constant8/1 -> Relational Operator8/1
  Relational Operator8/1 -> Switch8/2
  Relational Operator9/1 -> Switch9/2
  Constant9/1 -> Relational Operator9/1
  Md10Rsp/1 -> Relational Operator9/2, Switch9/1
  Switch9/1 -> Switch8/3
  Switch10/1 -> Switch9/3
  Md11Rsp/1 -> Relational Operator10/2, Switch10/1
  Constant10/1 -> Relational Operator10/1
  Relational Operator10/1 -> Switch10/2
  Relational Operator11/1 -> Switch11/2
  Constant11/1 -> Relational Operator11/1
  Md12Rsp/1 -> Relational Operator11/2, Switch11/1
  Switch11/1 -> Switch10/3
  Switch12/1 -> Switch11/3
  Md13Rsp/1 -> Relational Operator12/2, Switch12/1
  Constant12/1 -> Relational Operator12/1
  Relational Operator12/1 -> Switch12/2
  Relational Operator13/1 -> Switch13/2
  Constant13/1 -> Relational Operator13/1
  Md14Rsp/1 -> Relational Operator13/2, Switch13/1
  Switch13/1 -> Switch12/3
  Md21Rsp/1 -> Terminator_6/1
  Md22Rsp/1 -> Terminator_7/1
  Md23Rsp/1 -> Terminator_8/1
  Md24Rsp/1 -> Terminator_9/1
  Md25Rsp/1 -> Terminator_10/1
  Md26Rsp/1 -> Terminator_11/1
  Md27Rsp/1 -> Terminator_12/1
  Md28Rsp/1 -> Terminator_13/1
  Md29Rsp/1 -> Terminator_14/1
  Md30Rsp/1 -> Terminator_15/1
  Md31Rsp/1 -> Terminator_16/1
  Md32Rsp/1 -> Terminator_17/1
  Switch15/1 -> Switch14/3
  Md15Rsp/1 -> Switch14/1, Relational Operator14/2
  Constant14/1 -> Relational Operator14/1
  Relational Operator14/1 -> Switch14/2
  Switch14/1 -> Switch13/3
  Md16Rsp/1 -> Switch15/1, Relational Operator15/2
  Relational Operator15/1 -> Switch15/2
  Constant15/1 -> Relational Operator15/1
  Switch16/1 -> Switch15/3
  Switch17/1 -> Switch16/3
  Constant16/1 -> Relational Operator16/1
  Relational Operator16/1 -> Switch16/2
  Md17Rsp/1 -> Relational Operator16/2, Switch16/1
  Md18Rsp/1 -> Switch17/1, Relational Operator17/2
  Relational Operator17/1 -> Switch17/2
  Constant17/1 -> Relational Operator17/1
  Md20Rsp/1 -> Switch18/3
  Constant18/1 -> Relational Operator18/1
  Relational Operator18/1 -> Switch18/2
  Md19Rsp/1 -> Relational Operator18/2, Switch18/1
  Switch18/1 -> Switch17/3

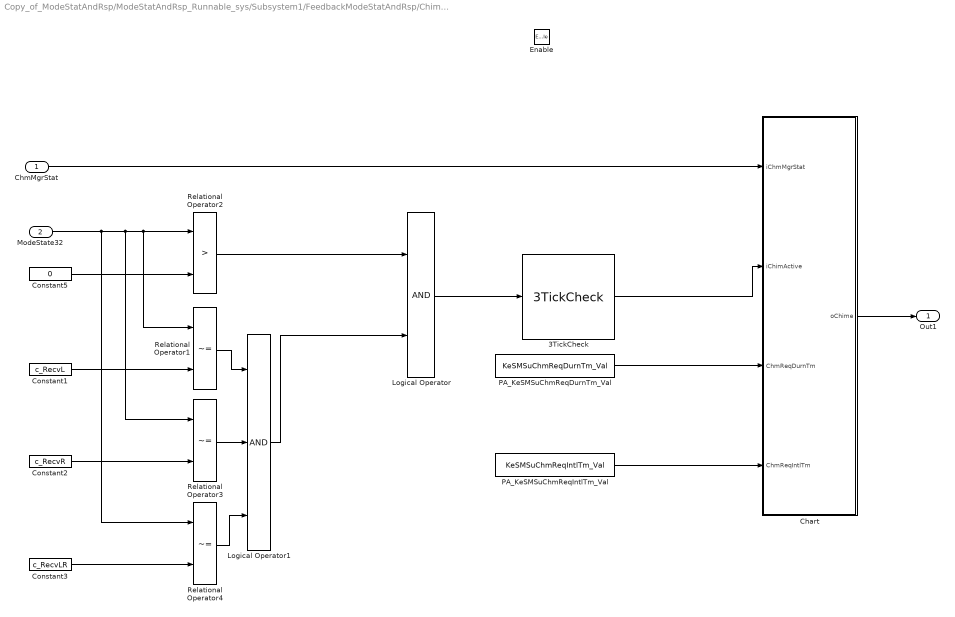
== system Copy_of_ModeStatAndRsp/ModeStatAndRsp_Runnable_sys/Subsystem1/FeedbackModeStatAndRsp/Chime2_3A6 ==
  ChmMgrStat : Inport
  ModeState32 : Inport  Port=2
  Enable : EnablePort
  3TickCheck : RspLib/3TickCheck  SystemSampleTime=-1
  Chart : Stateflow chart  TreatAsAtomicUnit=on
  Constant1 : Constant  Value=c_RecvL  OutDataTypeStr=uint32
  Constant2 : Constant  Value=c_RecvR  OutDataTypeStr=uint32
  Constant3 : Constant  Value=c_RecvLR  OutDataTypeStr=uint32
  Constant5 : Constant  Value=0  OutDataTypeStr=uint32
  Logical Operator : Logic  AllPortsSameDT=off  OutDataTypeStr=boolean
  Logical Operator1 : Logic  Inputs=3  AllPortsSameDT=off  OutDataTypeStr=boolean
  PA_KeSMSuChmReqDurnTm_Val : Constant  Value=KeSMSuChmReqDurnTm_Val
  PA_KeSMSuChmReqIntlTm_Val : Constant  Value=KeSMSuChmReqIntlTm_Val
  Relational Operator1 : RelationalOperator  Operator=~=  OutDataTypeStr=boolean  RndMeth=Simplest
  Relational Operator2 : RelationalOperator  Operator=>  OutDataTypeStr=boolean  RndMeth=Simplest
  Relational Operator3 : RelationalOperator  Operator=~=  OutDataTypeStr=boolean  RndMeth=Simplest
  Relational Operator4 : RelationalOperator  Operator=~=  OutDataTypeStr=boolean  RndMeth=Simplest
  Out1 : Outport
  wires:
  ChmMgrStat/1 -> Chart/1(iChmMgrStat)
  Chart/1(oChime) -> Out1/1
  3TickCheck/1 -> Chart/2(iChimActive)
  Constant5/1 -> Relational Operator2/2
  ModeState32/1 -> Relational Operator4/1, Relational Operator3/1, Relational Operator1/1, Relational Operator2/1
  Relational Operator2/1 -> Logical Operator/1
  Logical Operator/1 -> 3TickCheck/1
  Logical Operator1/1 -> Logical Operator/2
  Relational Operator1/1 -> Logical Operator1/1
  Relational Operator3/1 -> Logical Operator1/2
  Constant1/1 -> Relational Operator1/2
  Constant2/1 -> Relational Operator3/2
  Constant3/1 -> Relational Operator4/2
  Relational Operator4/1 -> Logical Operator1/3
  PA_KeSMSuChmReqDurnTm_Val/1 -> Chart/3(ChmReqDurnTm)
  PA_KeSMSuChmReqIntlTm_Val/1 -> Chart/4(ChmReqIntlTm)

== system Copy_of_ModeStatAndRsp/ModeStatAndRsp_Runnable_sys/Subsystem1/FeedbackModeStatAndRsp/FeedbackPassCmprtHMIDisCmd ==
  powerMode : Inport
  ModeState32 : Inport  Port=2
  3TickCheck : RspLib/3TickCheck  SystemSampleTime=-1
  Constant : Constant  Value=PowerMode1.PowerMode_Off  OutDataTypeStr=Enum:PowerMode1
  Constant2 : Constant  OutDataTypeStr=uint8
  Constant3 : Constant  Value=0  OutDataTypeStr=uint8
  Constant5 : Constant  Value=0  OutDataTypeStr=uint32
  Logical Operator : Logic  AllPortsSameDT=off  OutDataTypeStr=boolean
  Relational Operator1 : RelationalOperator  Operator===  OutDataTypeStr=boolean  RndMeth=Simplest
  Relational Operator2 : RelationalOperator  Operator=>  OutDataTypeStr=boolean  RndMeth=Simplest
  Switch : Switch  Criteria=u2 > Threshold
  StPassCmprtMdHMIDisCmd : Outport
  wires:
  powerMode/1 -> Relational Operator1/1
  Constant/1 -> Relational Operator1/2
  Switch/1 -> StPassCmprtMdHMIDisCmd/1
  Constant2/1 -> Switch/1
  Constant3/1 -> Switch/3
  Relational Operator1/1 -> Logical Operator/1
  Relational Operator2/1 -> Logical Operator/2
  Logical Operator/1 -> 3TickCheck/1
  3TickCheck/1 -> Switch/2
  ModeState32/1 -> Relational Operator2/1
  Constant5/1 -> Relational Operator2/2

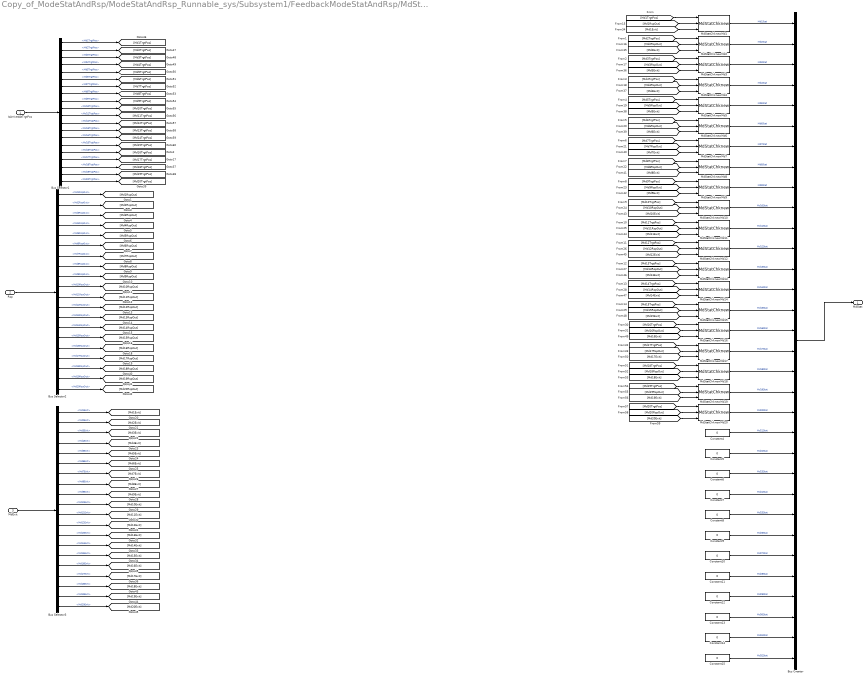
== system Copy_of_ModeStatAndRsp/ModeStatAndRsp_Runnable_sys/Subsystem1/FeedbackModeStatAndRsp/MdStatComm ==
  IsArrivedAtTrgtPos : Inport
  Rsp : Inport  Port=2
  MdExit : Inport  Port=3
  Bus Creator : BusCreator  Inputs=32
  Bus Selector1 : BusSelector  OutputSignals=Md1TrgtPos,Md2TrgtPos,Md3TrgtPos,Md4TrgtPos,Md5TrgtPos,Md6TrgtPos,Md7TrgtPos,Md8TrgtPos,Md9TrgtPos,Md10TrgtPos,Md11TrgtPos,Md12TrgtPos,Md13TrgtPos,Md14TrgtPos,Md15TrgtPos,Md16TrgtPos,Md17TrgtPos,Md18TrgtPos,Md19TrgtPos,Md20TrgtPos
  Bus Selector2 : BusSelector  OutputSignals=Md1RspOut,Md2RspOut,Md3RspOut,Md4RspOut,Md5RspOut,Md6RspOut,Md7RspOut,Md8RspOut,Md9RspOut,Md10RspOut,Md11RspOut,Md12RspOut,Md13RspOut,Md14RspOut,Md15RspOut,Md16RspOut,Md17RspOut,Md18RspOut,Md19RspOut,Md20RspOut
  Bus Selector3 : BusSelector  OutputSignals=Md1Exit,Md2Exit,Md3Exit,Md4Exit,Md5Exit,Md6Exit,Md7Exit,Md8Exit,Md9Exit,Md10Exit,Md11Exit,Md12Exit,Md13Exit,Md14Exit,Md15Exit,Md16Exit,Md17Exit,Md18Exit,Md19Exit,Md20Exit
  Constant{4..15} (12 alike) : Constant  Value=0  OutDataTypeStr=uint8
  MdStatChknewMd{1..20} (20 alike) : RspLib/MdStatChknew  SystemSampleTime=-1
  MdStat : Outport
  wires:
  IsArrivedAtTrgtPos/1 -> Bus Selector1/1
  Bus Selector1/5 -> [Md5TrgtPos]  "<Md5TrgtPos>"
  Bus Selector1/6 -> [Md6TrgtPos]  "<Md6TrgtPos>"
  Bus Selector1/1 -> [Md1TrgtPos]  "<Md1TrgtPos>"
  Bus Selector1/4 -> [Md4TrgtPos]  "<Md4TrgtPos>"
  Bus Selector1/2 -> [Md2TrgtPos]  "<Md2TrgtPos>"
  Bus Selector1/3 -> [Md3TrgtPos]  "<Md3TrgtPos>"
  Bus Selector1/10 -> [Md10TrgtPos]  "<Md10TrgtPos>"
  Bus Selector1/11 -> [Md11TrgtPos]  "<Md11TrgtPos>"
  Bus Selector1/8 -> [Md8TrgtPos]  "<Md8TrgtPos>"
  Bus Selector1/12 -> [Md12TrgtPos]  "<Md12TrgtPos>"
  Bus Selector1/7 -> [Md7TrgtPos]  "<Md7TrgtPos>"
  Bus Selector1/9 -> [Md9TrgtPos]  "<Md9TrgtPos>"
  Bus Selector1/14 -> [Md14TrgtPos]  "<Md14TrgtPos>"
  Bus Selector1/13 -> [Md13TrgtPos]  "<Md13TrgtPos>"
  Bus Selector1/15 -> [Md15TrgtPos]  "<Md15TrgtPos>"
  Rsp/1 -> Bus Selector2/1
  Bus Selector2/6 -> [Md6RspOut]  "<Md6RspOut>"
  Bus Selector2/15 -> [Md15RspOut]  "<Md15RspOut>"
  Bus Selector2/1 -> [Md1RspOut]  "<Md1RspOut>"
  Bus Selector2/14 -> [Md14RspOut]  "<Md14RspOut>"
  Bus Selector2/5 -> [Md5RspOut]  "<Md5RspOut>"
  Bus Selector2/2 -> [Md2RspOut]  "<Md2RspOut>"
  Bus Selector2/8 -> [Md8RspOut]  "<Md8RspOut>"
  Bus Selector2/3 -> [Md3RspOut]  "<Md3RspOut>"
  Bus Selector2/9 -> [Md9RspOut]  "<Md9RspOut>"
  Bus Selector2/7 -> [Md7RspOut]  "<Md7RspOut>"
  Bus Selector2/11 -> [Md11RspOut]  "<Md11RspOut>"
  Bus Selector2/12 -> [Md12RspOut]  "<Md12RspOut>"
  Bus Selector2/13 -> [Md13RspOut]  "<Md13RspOut>"
  Bus Selector2/10 -> [Md10RspOut]  "<Md10RspOut>"
  Bus Selector2/4 -> [Md4RspOut]  "<Md4RspOut>"
  Bus Creator/1 -> MdStat/1
  MdStatChknewMd1/1 -> Bus Creator/1  "Md1Stat"
  [Md1TrgtPos] -> MdStatChknewMd1/1
  [Md1RspOut] -> MdStatChknewMd1/2
  MdStatChknewMd2/1 -> Bus Creator/2  "Md2Stat"
  [Md2TrgtPos] -> MdStatChknewMd2/1
  MdStatChknewMd3/1 -> Bus Creator/3  "Md3Stat"
  MdStatChknewMd4/1 -> Bus Creator/4  "Md4Stat"
  MdStatChknewMd5/1 -> Bus Creator/5  "Md5Stat"
  MdStatChknewMd6/1 -> Bus Creator/6  "Md6Stat"
  MdStatChknewMd7/1 -> Bus Creator/7  "Md7Stat"
  MdStatChknewMd8/1 -> Bus Creator/8  "Md8Stat"
  MdStatChknewMd9/1 -> Bus Creator/9  "Md9Stat"
  MdStatChknewMd10/1 -> Bus Creator/10  "Md10Stat"
  MdStatChknewMd11/1 -> Bus Creator/11  "Md11Stat"
  MdStatChknewMd12/1 -> Bus Creator/12  "Md12Stat"
  MdStatChknewMd13/1 -> Bus Creator/13  "Md13Stat"
  MdStatChknewMd14/1 -> Bus Creator/14  "Md14Stat"
  MdStatChknewMd15/1 -> Bus Creator/15  "Md15Stat"
  MdStatChknewMd16/1 -> Bus Creator/16  "Md16Stat"
  MdStatChknewMd17/1 -> Bus Creator/17  "Md17Stat"
  MdStatChknewMd18/1 -> Bus Creator/18  "Md18Stat"
  MdStatChknewMd19/1 -> Bus Creator/19  "Md19Stat"
  MdStatChknewMd20/1 -> Bus Creator/20  "Md20Stat"
  Constant4/1 -> Bus Creator/21  "Md21Stat"
  Constant5/1 -> Bus Creator/22  "Md22Stat"
  Constant6/1 -> Bus Creator/23  "Md23Stat"
  Constant7/1 -> Bus Creator/24  "Md24Stat"
  Constant8/1 -> Bus Creator/25  "Md25Stat"
  Constant9/1 -> Bus Creator/26  "Md26Stat"
  Constant10/1 -> Bus Creator/27  "Md27Stat"
  Constant12/1 -> Bus Creator/29  "Md29Stat"
  Constant11/1 -> Bus Creator/28  "Md28Stat"
  Constant13/1 -> Bus Creator/30  "Md30Stat"
  Constant14/1 -> Bus Creator/31  "Md31Stat"
  Constant15/1 -> Bus Creator/32  "Md32Stat"
  [Md3TrgtPos] -> MdStatChknewMd3/1
  [Md4TrgtPos] -> MdStatChknewMd4/1
  [Md5TrgtPos] -> MdStatChknewMd5/1
  [Md6TrgtPos] -> MdStatChknewMd6/1
  [Md7TrgtPos] -> MdStatChknewMd7/1
  [Md8TrgtPos] -> MdStatChknewMd8/1
  [Md9TrgtPos] -> MdStatChknewMd9/1
  [Md10TrgtPos] -> MdStatChknewMd10/1
  [Md11TrgtPos] -> MdStatChknewMd11/1
  [Md12TrgtPos] -> MdStatChknewMd12/1
  [Md13TrgtPos] -> MdStatChknewMd13/1
  [Md14TrgtPos] -> MdStatChknewMd14/1
  [Md15TrgtPos] -> MdStatChknewMd15/1
  [Md2RspOut] -> MdStatChknewMd2/2
  [Md3RspOut] -> MdStatChknewMd3/2
  [Md4RspOut] -> MdStatChknewMd4/2
  [Md5RspOut] -> MdStatChknewMd5/2
  [Md6RspOut] -> MdStatChknewMd6/2
  [Md7RspOut] -> MdStatChknewMd7/2
  [Md9RspOut] -> MdStatChknewMd9/2
  [Md10RspOut] -> MdStatChknewMd10/2
  [Md13RspOut] -> MdStatChknewMd13/2
  [Md14RspOut] -> MdStatChknewMd14/2
  [Md15RspOut] -> MdStatChknewMd15/2
  Bus Selector1/17 -> [Md17TrgtPos]  "<Md17TrgtPos>"
  Bus Selector1/16 -> [Md16TrgtPos]  "<Md16TrgtPos>"
  Bus Selector2/16 -> [Md16RspOut]  "<Md16RspOut>"
  Bus Selector2/17 -> [Md17RspOut]  "<Md17RspOut>"
  [Md16TrgtPos] -> MdStatChknewMd16/1
  [Md17TrgtPos] -> MdStatChknewMd17/1
  [Md8RspOut] -> MdStatChknewMd8/2
  [Md11RspOut] -> MdStatChknewMd11/2
  [Md12RspOut] -> MdStatChknewMd12/2
  [Md16RspOut] -> MdStatChknewMd16/2
  [Md17RspOut] -> MdStatChknewMd17/2
  MdExit/1 -> Bus Selector3/1
  Bus Selector3/1 -> [Md1Exit]  "<Md1Exit>"
  Bus Selector3/2 -> [Md2Exit]  "<Md2Exit>"
  Bus Selector3/3 -> [Md3Exit]  "<Md3Exit>"
  Bus Selector3/4 -> [Md4Exit]  "<Md4Exit>"
  Bus Selector3/5 -> [Md5Exit]  "<Md5Exit>"
  Bus Selector3/6 -> [Md6Exit]  "<Md6Exit>"
  Bus Selector3/7 -> [Md7Exit]  "<Md7Exit>"
  Bus Selector3/8 -> [Md8Exit]  "<Md8Exit>"
  Bus Selector3/9 -> [Md9Exit]  "<Md9Exit>"
  Bus Selector3/10 -> [Md10Exit]  "<Md10Exit>"
  Bus Selector3/11 -> [Md11Exit]  "<Md11Exit>"
  Bus Selector3/12 -> [Md12Exit]  "<Md12Exit>"
  Bus Selector3/13 -> [Md13Exit]  "<Md13Exit>"
  Bus Selector3/14 -> [Md14Exit]  "<Md14Exit>"
  Bus Selector3/15 -> [Md15Exit]  "<Md15Exit>"
  Bus Selector3/16 -> [Md16Exit]  "<Md16Exit>"
  Bus Selector3/17 -> [Md17Exit]  "<Md17Exit>"
  [Md1Exit] -> MdStatChknewMd1/3
  [Md2Exit] -> MdStatChknewMd2/3
  [Md3Exit] -> MdStatChknewMd3/3
  [Md4Exit] -> MdStatChknewMd4/3
  [Md5Exit] -> MdStatChknewMd5/3
  [Md6Exit] -> MdStatChknewMd6/3
  [Md7Exit] -> MdStatChknewMd7/3
  [Md8Exit] -> MdStatChknewMd8/3
  [Md9Exit] -> MdStatChknewMd9/3
  [Md10Exit] -> MdStatChknewMd10/3
  [Md11Exit] -> MdStatChknewMd11/3
  [Md12Exit] -> MdStatChknewMd12/3
  [Md13Exit] -> MdStatChknewMd13/3
  [Md14Exit] -> MdStatChknewMd14/3
  [Md15Exit] -> MdStatChknewMd15/3
  [Md16Exit] -> MdStatChknewMd16/3
  [Md17Exit] -> MdStatChknewMd17/3
  [Md18Exit] -> MdStatChknewMd18/3
  [Md18RspOut] -> MdStatChknewMd18/2
  [Md18TrgtPos] -> MdStatChknewMd18/1
  [Md19TrgtPos] -> MdStatChknewMd19/1
  [Md19RspOut] -> MdStatChknewMd19/2
  [Md19Exit] -> MdStatChknewMd19/3
  [Md20Exit] -> MdStatChknewMd20/3
  [Md20RspOut] -> MdStatChknewMd20/2
  [Md20TrgtPos] -> MdStatChknewMd20/1
  Bus Selector1/18 -> [Md18TrgtPos]  "<Md18TrgtPos>"
  Bus Selector1/19 -> [Md19TrgtPos]  "<Md19TrgtPos>"
  Bus Selector1/20 -> [Md20TrgtPos]  "<Md20TrgtPos>"
  Bus Selector2/18 -> [Md18RspOut]  "<Md18RspOut>"
  Bus Selector2/19 -> [Md19RspOut]  "<Md19RspOut>"
  Bus Selector2/20 -> [Md20RspOut]  "<Md20RspOut>"
  Bus Selector3/18 -> [Md18Exit]  "<Md18Exit>"
  Bus Selector3/19 -> [Md19Exit]  "<Md19Exit>"
  Bus Selector3/20 -> [Md20Exit]  "<Md20Exit>"
